simulink model "FBv1_SLOW2DOF"  (R2022b)
settings: Solver=FixedStepAuto  StartTime=0.0  StopTime=Parameter.Time.TMax  FixedStep=Parameter.Time.dt  RelTol=1e-3
values from neighbouring files (symbols this model uses):
  Parameter = DefaultParameter_FBv1_ADv14(Parameter)    [Turbine_Simulation.m]
undefined symbols (not defined in the file or in its folder): x2_t0
libraries: simulink x4
settings Model: LastModifiedBy=felix
settings OptimizationCC: BlockReduction=off  BooleanDataType=off
settings DebuggingCC: SaveWithParameterizedLinksMsg=none  UnderspecifiedInitializationDetection=Classic  MergeDetectMultiDrivingBlocksExec=none  SignalResolutionControl=TryResolveAllWithWarning
settings HardwareCC: TargetUnknown=on
settings ModelReferenceCC: PropagateSignalLabelsOutOfModel=off

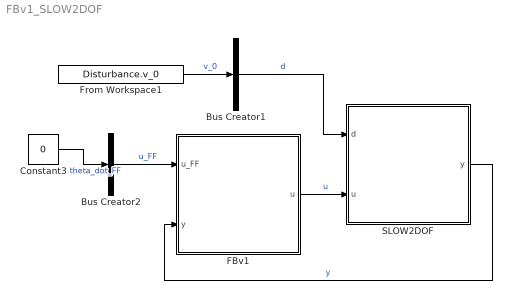
== system FBv1_SLOW2DOF ==
  Bus Creator1 : BusCreator  Inputs=1
  Bus Creator2 : BusCreator  Inputs=1
  Constant3 : Constant  Value=0
  FBv1 : Subsystem
  From Workspace1 : FromWorkspace  VariableName=Disturbance.v_0
  SLOW2DOF : Subsystem
  wires:
  FBv1/1(u) -> SLOW2DOF/2(u)  "u"
  Bus Creator2/1 -> FBv1/1(u_FF)  "u_FF"
  Bus Creator1/1 -> SLOW2DOF/1(d)  "d"
  From Workspace1/1 -> Bus Creator1/1  "v_0"
  SLOW2DOF/1(y) -> FBv1/2(y)  "y"
  Constant3/1 -> Bus Creator2/1  "theta_dot_FF"

== system FBv1_SLOW2DOF/FBv1 ==
  u_FF : Inport
  y : Inport  Port=2
  Bus Creator1 : BusCreator  Inputs=2
  Bus Selector : BusSelector  OutputSignals=Omega_g
  Bus Selector1 : BusSelector  OutputSignals=theta
  Bus Selector2 : BusSelector  OutputSignals=M_g
  FBv1 : Subsystem
  Terminator : Terminator
  u : Outport
  wires:
  y/1 -> Bus Selector2/1, Bus Selector1/1, Bus Selector/1  "y"
  Bus Creator1/1 -> u/1  "u"
  Bus Selector/1 -> FBv1/1(Omega_g [rad/s])  "<Omega_g>"
  u_FF/1 -> Terminator/1
  Bus Selector1/1 -> FBv1/3(theta [rad])  "<theta>"
  FBv1/1(M_g_c [Nm]) -> Bus Creator1/1  "M_g_c"
  FBv1/2(theta_c [rad]) -> Bus Creator1/2  "theta_c"
  Bus Selector2/1 -> FBv1/2(M_g [Nm])  "<M_g>"

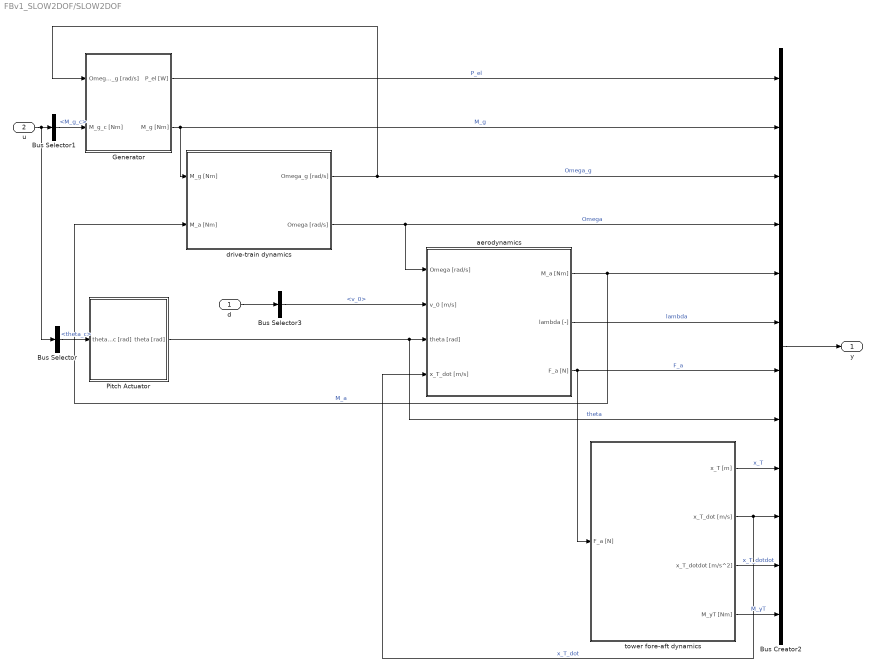
== system FBv1_SLOW2DOF/SLOW2DOF ==
  d : Inport
  u : Inport  Port=2
  Bus Creator2 : BusCreator  Inputs=12
  Bus Selector : BusSelector  OutputSignals=theta_c
  Bus Selector1 : BusSelector  OutputSignals=M_g_c
  Bus Selector3 : BusSelector  OutputSignals=v_0
  Generator : Subsystem
  Pitch Actuator : Subsystem
  "aerodynamics " : Subsystem
  drive-train dynamics : Subsystem
  tower fore-aft dynamics : Subsystem
  y : Outport
  wires:
  Bus Selector3/1 -> "aerodynamics "/2(v_0 [m/s])  "<v_0>"
  d/1 -> Bus Selector3/1
  "aerodynamics "/2(lambda [-]) -> Bus Creator2/6  "lambda"
  Bus Selector/1 -> Pitch Actuator/1(theta_c [rad])  "<theta_c>"
  u/1 -> Bus Selector/1, Bus Selector1/1
  "aerodynamics "/1(M_a [Nm]) -> Bus Creator2/5, drive-train dynamics/2(M_a [Nm])  "M_a"
  drive-train dynamics/2(Omega [rad/s]) -> Bus Creator2/4, "aerodynamics "/1(Omega [rad/s])  "Omega"
  drive-train dynamics/1(Omega_g [rad/s]) -> Bus Creator2/3, Generator/1(Omega_g [rad/s])  "Omega_g"
  Bus Selector1/1 -> Generator/2(M_g_c [Nm])  "<M_g_c>"
  Pitch Actuator/1(theta [rad]) -> Bus Creator2/8, "aerodynamics "/3(theta [rad])  "theta"
  Generator/1(P_el [W]) -> Bus Creator2/1  "P_el"
  Generator/2(M_g [Nm]) -> Bus Creator2/2, drive-train dynamics/1(M_g [Nm])  "M_g"
  "aerodynamics "/3(F_a [N]) -> Bus Creator2/7, tower fore-aft dynamics/1(F_a [N])  "F_a"
  tower fore-aft dynamics/1(x_T [m]) -> Bus Creator2/9  "x_T"
  tower fore-aft dynamics/2(x_T_dot [m/s]) -> "aerodynamics "/4(x_T_dot [m/s]), Bus Creator2/10  "x_T_dot"
  tower fore-aft dynamics/3(x_T_dotdot [m/s^2]) -> Bus Creator2/11  "x_T_dotdot"
  tower fore-aft dynamics/4(M_yT [Nm]) -> Bus Creator2/12  "M_yT"
  Bus Creator2/1 -> y/1

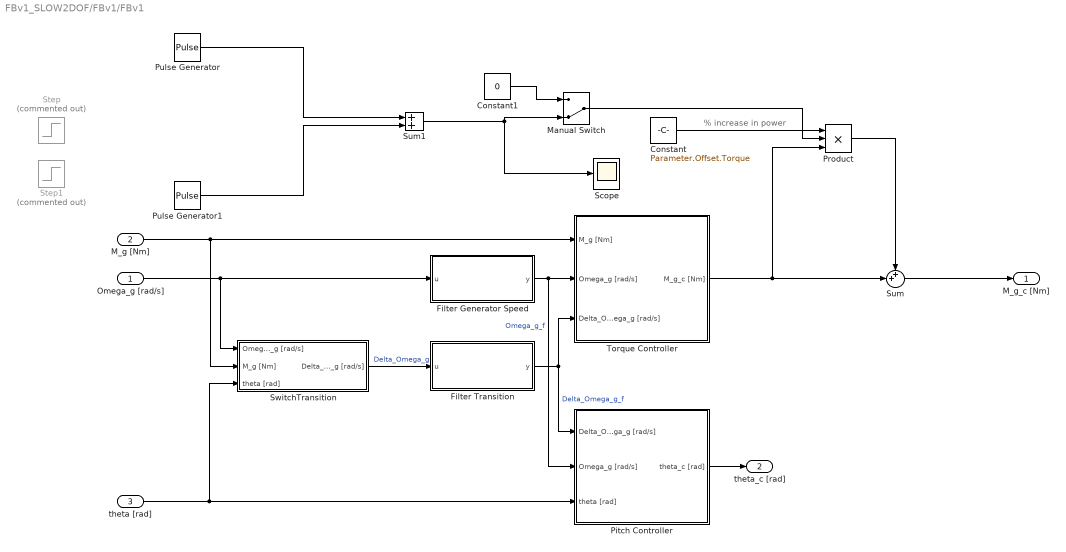
== system FBv1_SLOW2DOF/FBv1/FBv1 ==
  note: % increase in power
  Omega_g [rad/s] : Inport
  M_g [Nm] : Inport  Port=2
  theta [rad] : Inport  Port=3
  Constant : Constant  Value=Parameter.Offset.Torque
  Constant1 : Constant  Value=0
  Filter Generator Speed : Subsystem
  Filter Transition : Subsystem
  Manual Switch : ManualSwitch  CurrentSetting=0
  Pitch Controller : Subsystem
  Product : Product  Inputs=3
  Pulse Generator : DiscretePulseGenerator  PulseType=Time based  Period=Parameter.Offset.positive.period  PulseWidth=Parameter.Offset.positive.width  PhaseDelay=Parameter.Offset.positive.delay
  Pulse Generator1 : DiscretePulseGenerator  PulseType=Time based  Amplitude=-1  Period=Parameter.Offset.negative.period  PulseWidth=Parameter.Offset.negative.width  PhaseDelay=Parameter.Offset.negative.delay
  Scope : Scope
  Step : Step  Commented=on  Time=30  SampleTime=0
  Step1 : Step  Commented=on  Time=32  Before=1  After=0  SampleTime=0
  Sum : Sum  Inputs=++|
  Sum1 : Sum
  SwitchTransition : Subsystem
  Torque Controller : Subsystem
  M_g_c [Nm] : Outport
  theta_c [rad] : Outport  Port=2
  wires:
  Pitch Controller/1(theta_c [rad]) -> theta_c [rad]/1
  Omega_g [rad/s]/1 -> SwitchTransition/1(Omega_g [rad/s]), Filter Generator Speed/1(u)
  SwitchTransition/1(Delta_Omega_g [rad/s]) -> Filter Transition/1(u)  "Delta_Omega_g"
  Filter Transition/1(y) -> Pitch Controller/1(Delta_Omega_g [rad/s]), Torque Controller/3(Delta_Omega_g [rad/s])  "Delta_Omega_g_f"
  Filter Generator Speed/1(y) -> Torque Controller/2(Omega_g [rad/s]), Pitch Controller/2(Omega_g [rad/s])  "Omega_g_f"
  theta [rad]/1 -> Pitch Controller/3(theta [rad]), SwitchTransition/3(theta [rad])
  M_g [Nm]/1 -> SwitchTransition/2(M_g [Nm]), Torque Controller/1(M_g [Nm])
  Torque Controller/1(M_g_c [Nm]) -> Sum/2, Product/3
  Sum/1 -> M_g_c [Nm]/1
  Constant/1 -> Product/1
  Product/1 -> Sum/1
  Manual Switch/1 -> Product/2
  Constant1/1 -> Manual Switch/1
  Sum1/1 -> Scope/1, Manual Switch/2
  Pulse Generator1/1 -> Sum1/2
  Pulse Generator/1 -> Sum1/1

== system FBv1_SLOW2DOF/SLOW2DOF/Generator ==
  Omega_g [rad/s] : Inport
  M_g_c [Nm] : Inport  Port=2
  Constant3 : Constant  Value=Parameter.Generator.eta_el
  Product1 : Product  Inputs=***  RndMeth=Zero
  Simple Torque Actuator : Memory  InitialCondition=Parameter.IC.M_g
  P_el [W] : Outport
  M_g [Nm] : Outport  Port=2
  wires:
  Constant3/1 -> Product1/3
  M_g_c [Nm]/1 -> Simple Torque Actuator/1
  Omega_g [rad/s]/1 -> Product1/2
  Product1/1 -> P_el [W]/1
  Simple Torque Actuator/1 -> M_g [Nm]/1, Product1/1

== system FBv1_SLOW2DOF/SLOW2DOF/Pitch Actuator ==
  theta_c [rad] : Inport
  Constant2 : Constant  Value=Parameter.IC.theta
  PT2 : Subsystem  mask{omega=Parameter.PitchActuator.omega, xi=Parameter.PitchActuator.xi, x1_max=Parameter.PitchActuator.theta_dot_max, x1_min=-Parameter.PitchActuator.theta_dot_max, x2_max=Parameter.PitchActuator.theta_max, x2_min=Parameter.PitchActuator.theta_min}
      mask prompts: omega "undamped natural frequency [rad/s]"; xi "damping factor [-]"; x1_max "Upper bound x1"; x1_min "Lower bound x1"; x2_max "Upper bound x2"; x2_min "Lower bound x2"
      mask Display:
      | disp(['omega = ',num2str(omega),'\n'...
      |     ,'xi = ',num2str(xi)])
      | port_label('output',1,'y')
      | port_label('output',2,'x1')
      | port_label('input',2,'y0')
      | port_label('input',1,'u')
  Terminator : Terminator
  theta [rad] : Outport
  wires:
  theta_c [rad]/1 -> PT2/1(u)
  Constant2/1 -> PT2/2(y0)
  PT2/1(y) -> theta [rad]/1
  PT2/2(x1) -> Terminator/1

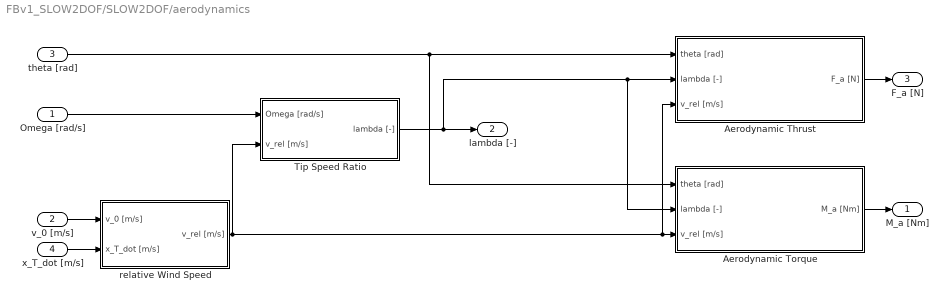
== system FBv1_SLOW2DOF/SLOW2DOF/aerodynamics  ==
  Omega [rad/s] : Inport
  v_0 [m/s] : Inport  Port=2
  theta [rad] : Inport  Port=3
  x_T_dot [m/s] : Inport  Port=4
  Aerodynamic Thrust : Subsystem
  Aerodynamic Torque : Subsystem
  Tip Speed Ratio : Subsystem
  relative Wind Speed : Subsystem
  M_a [Nm] : Outport
  lambda [-] : Outport  Port=2
  F_a [N] : Outport  Port=3
  wires:
  theta [rad]/1 -> Aerodynamic Thrust/1(theta [rad]), Aerodynamic Torque/1(theta [rad])
  Aerodynamic Torque/1(M_a [Nm]) -> M_a [Nm]/1
  Aerodynamic Thrust/1(F_a [N]) -> F_a [N]/1
  x_T_dot [m/s]/1 -> relative Wind Speed/2(x_T_dot [m/s])
  v_0 [m/s]/1 -> relative Wind Speed/1(v_0 [m/s])
  Omega [rad/s]/1 -> Tip Speed Ratio/1(Omega [rad/s])
  relative Wind Speed/1(v_rel [m/s]) -> Tip Speed Ratio/2(v_rel [m/s]), Aerodynamic Torque/3(v_rel [m/s]), Aerodynamic Thrust/3(v_rel [m/s])
  Tip Speed Ratio/1(lambda [-]) -> Aerodynamic Thrust/2(lambda [-]), Aerodynamic Torque/2(lambda [-]), lambda [-]/1

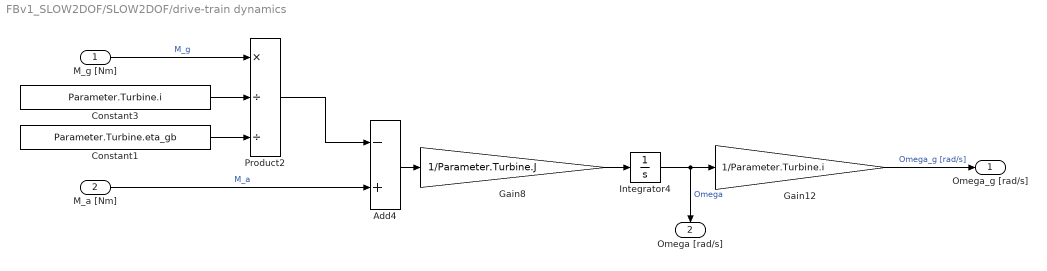
== system FBv1_SLOW2DOF/SLOW2DOF/drive-train dynamics ==
  M_g [Nm] : Inport
  M_a [Nm] : Inport  Port=2
  Add4 : Sum  Inputs=-+
  Constant1 : Constant  Value=Parameter.Turbine.eta_gb
  Constant3 : Constant  Value=Parameter.Turbine.i
  Gain12 : Gain  Gain=1/Parameter.Turbine.i  SaturateOnIntegerOverflow=on  OutDataTypeStr=Inherit: Same as input  ParamDataTypeStr=Inherit: Same as input
  Gain8 : Gain  Gain=1/Parameter.Turbine.J  SaturateOnIntegerOverflow=on  OutDataTypeStr=Inherit: Same as input  ParamDataTypeStr=Inherit: Same as input
  Integrator4 : Integrator  InitialCondition=Parameter.IC.Omega
  Product2 : Product  Inputs=*//  RndMeth=Zero
  Omega_g [rad/s] : Outport
  Omega [rad/s] : Outport  Port=2
  wires:
  M_a [Nm]/1 -> Add4/2  "M_a"
  Integrator4/1 -> Omega [rad/s]/1, Gain12/1  "Omega"
  Add4/1 -> Gain8/1
  Gain8/1 -> Integrator4/1
  Product2/1 -> Add4/1
  Gain12/1 -> Omega_g [rad/s]/1  "Omega_g [rad/s]"
  M_g [Nm]/1 -> Product2/1  "M_g"
  Constant3/1 -> Product2/2
  Constant1/1 -> Product2/3

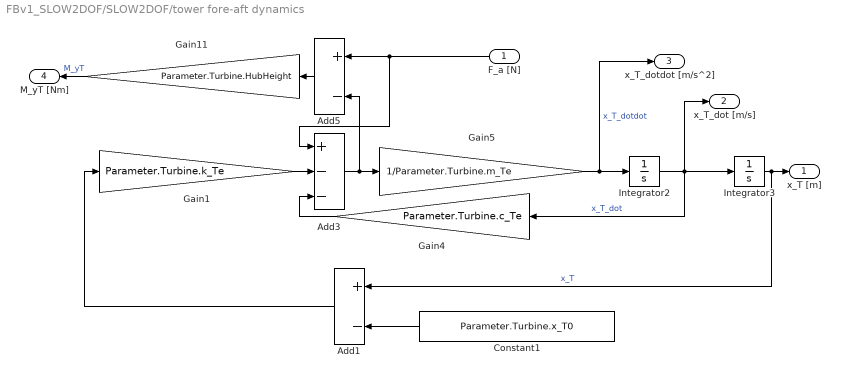
== system FBv1_SLOW2DOF/SLOW2DOF/tower fore-aft dynamics ==
  F_a [N] : Inport
  Add1 : Sum  Inputs=+-
  Add3 : Sum  Inputs=+--
  Add5 : Sum  Inputs=+-
  Constant1 : Constant  Value=Parameter.Turbine.x_T0
  Gain1 : Gain  Gain=Parameter.Turbine.k_Te  SaturateOnIntegerOverflow=on  OutDataTypeStr=Inherit: Same as input  ParamDataTypeStr=Inherit: Same as input
  Gain11 : Gain  Gain=Parameter.Turbine.HubHeight  SaturateOnIntegerOverflow=on  OutDataTypeStr=Inherit: Same as input  ParamDataTypeStr=Inherit: Same as input
  Gain4 : Gain  Gain=Parameter.Turbine.c_Te  SaturateOnIntegerOverflow=on  OutDataTypeStr=Inherit: Same as input  ParamDataTypeStr=Inherit: Same as input
  Gain5 : Gain  Gain=1/Parameter.Turbine.m_Te  SaturateOnIntegerOverflow=on  OutDataTypeStr=Inherit: Same as input  ParamDataTypeStr=Inherit: Same as input
  Integrator2 : Integrator
  Integrator3 : Integrator  InitialCondition=Parameter.IC.x_T
  x_T [m] : Outport
  x_T_dot [m/s] : Outport  Port=2
  x_T_dotdot [m/s^2] : Outport  Port=3
  M_yT [Nm] : Outport  Port=4
  wires:
  Constant1/1 -> Add1/2
  Add1/1 -> Gain1/1
  Add3/1 -> Gain5/1, Add5/2
  Integrator2/1 -> Gain4/1, Integrator3/1, x_T_dot [m/s]/1  "x_T_dot"
  Integrator3/1 -> x_T [m]/1, Add1/1  "x_T"
  Gain4/1 -> Add3/3
  Gain1/1 -> Add3/2
  Gain5/1 -> x_T_dotdot [m/s^2]/1, Integrator2/1  "x_T_dotdot"
  Add5/1 -> Gain11/1
  Gain11/1 -> M_yT [Nm]/1  "M_yT"
  F_a [N]/1 -> Add5/1, Add3/1

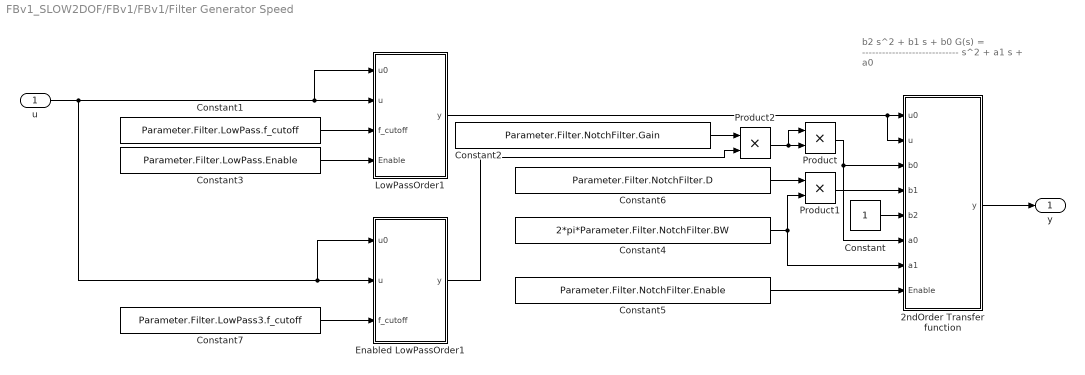
== system FBv1_SLOW2DOF/FBv1/FBv1/Filter Generator Speed ==
  note: b2 s^2 + b1 s + b0
      | G(s) = -----------------------------
      | s^2 + a1 s + a0
  u : Inport
  2ndOrder Transfer function : Subsystem
  Constant : Constant
  Constant1 : Constant  Value=Parameter.Filter.LowPass.f_cutoff
  Constant2 : Constant  Value=Parameter.Filter.NotchFilter.Gain
  Constant3 : Constant  Value=Parameter.Filter.LowPass.Enable
  Constant4 : Constant  Value=2*pi*Parameter.Filter.NotchFilter.BW
  Constant5 : Constant  Value=Parameter.Filter.NotchFilter.Enable
  Constant6 : Constant  Value=Parameter.Filter.NotchFilter.D
  Constant7 : Constant  Value=Parameter.Filter.LowPass3.f_cutoff
  Enabled LowPassOrder1 : Subsystem
  LowPassOrder1 : Subsystem
  Product : Product  RndMeth=Zero
  Product1 : Product  RndMeth=Zero
  Product2 : Product  RndMeth=Zero
  y : Outport
  wires:
  u/1 -> LowPassOrder1/1(u0), LowPassOrder1/2(u), Enabled LowPassOrder1/1(u0), Enabled LowPassOrder1/2(u)
  Constant3/1 -> LowPassOrder1/4(Enable)
  Constant1/1 -> LowPassOrder1/3(f_cutoff)
  LowPassOrder1/1(y) -> 2ndOrder Transfer function/2(u), 2ndOrder Transfer function/1(u0)
  Constant5/1 -> 2ndOrder Transfer function/8(Enable)
  Product/1 -> 2ndOrder Transfer function/3(b0), 2ndOrder Transfer function/6(a0)
  Product2/1 -> Product/1, Product/2
  Product1/1 -> 2ndOrder Transfer function/4(b1)
  Constant6/1 -> Product1/1
  Constant4/1 -> 2ndOrder Transfer function/7(a1), Product1/2
  2ndOrder Transfer function/1(y) -> y/1
  Constant/1 -> 2ndOrder Transfer function/5(b2)
  Constant7/1 -> Enabled LowPassOrder1/3(f_cutoff)
  Constant2/1 -> Product2/1
  Enabled LowPassOrder1/1(y) -> Product2/2

== system FBv1_SLOW2DOF/FBv1/FBv1/Filter Transition ==
  u : Inport
  Constant1 : Constant  Value=Parameter.Filter.LowPass2.f_cutoff
  Dummy : Constant  Value=0
  LowPassOrder1 : Subsystem
  y : Outport
  wires:
  LowPassOrder1/1(y) -> y/1
  u/1 -> LowPassOrder1/2(u)
  Constant1/1 -> LowPassOrder1/3(f_cutoff)
  Dummy/1 -> LowPassOrder1/1(u0)

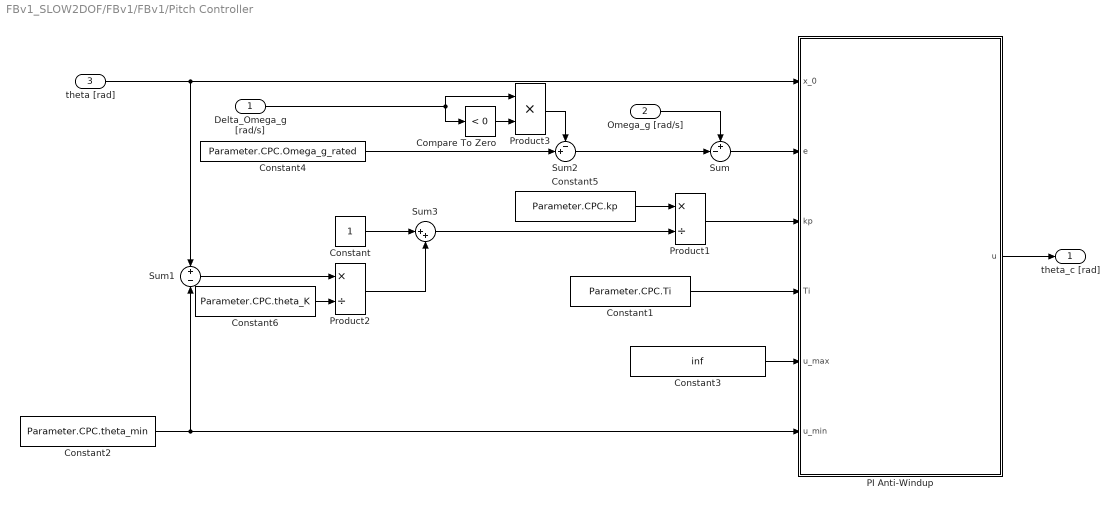
== system FBv1_SLOW2DOF/FBv1/FBv1/Pitch Controller ==
  Delta_Omega_g [rad/s] : Inport
  Omega_g [rad/s] : Inport  Port=2
  theta [rad] : Inport  Port=3
  Compare To Zero : simulink/Logic and Bit Operations/Compare To Zero  relop=<  OutDataTypeStr=boolean
  Constant : Constant
  Constant1 : Constant  Value=Parameter.CPC.Ti
  Constant2 : Constant  Value=Parameter.CPC.theta_min
  Constant3 : Constant  Value=inf
  Constant4 : Constant  Value=Parameter.CPC.Omega_g_rated
  Constant5 : Constant  Value=Parameter.CPC.kp
  Constant6 : Constant  Value=Parameter.CPC.theta_K
  PI Anti-Windup : Subsystem
  Product1 : Product  Inputs=*/
  Product2 : Product  Inputs=*/
  Product3 : Product
  Sum : Sum  Inputs=+-|
  Sum1 : Sum  Inputs=+|-
  Sum2 : Sum  Inputs=-+|
  Sum3 : Sum  Inputs=|++
  theta_c [rad] : Outport
  wires:
  Product1/1 -> PI Anti-Windup/3(kp)
  theta [rad]/1 -> PI Anti-Windup/1(x_0), Sum1/1
  Sum/1 -> PI Anti-Windup/2(e)
  PI Anti-Windup/1(u) -> theta_c [rad]/1
  Constant2/1 -> PI Anti-Windup/6(u_min), Sum1/2
  Delta_Omega_g [rad/s]/1 -> Product3/1, Compare To Zero/1
  Compare To Zero/1 -> Product3/2
  Product3/1 -> Sum2/1
  Constant4/1 -> Sum2/2
  Constant1/1 -> PI Anti-Windup/4(Ti)
  Sum2/1 -> Sum/2
  Omega_g [rad/s]/1 -> Sum/1
  Constant3/1 -> PI Anti-Windup/5(u_max)
  Sum1/1 -> Product2/1
  Constant6/1 -> Product2/2
  Constant/1 -> Sum3/1
  Product2/1 -> Sum3/2
  Constant5/1 -> Product1/1
  Sum3/1 -> Product1/2

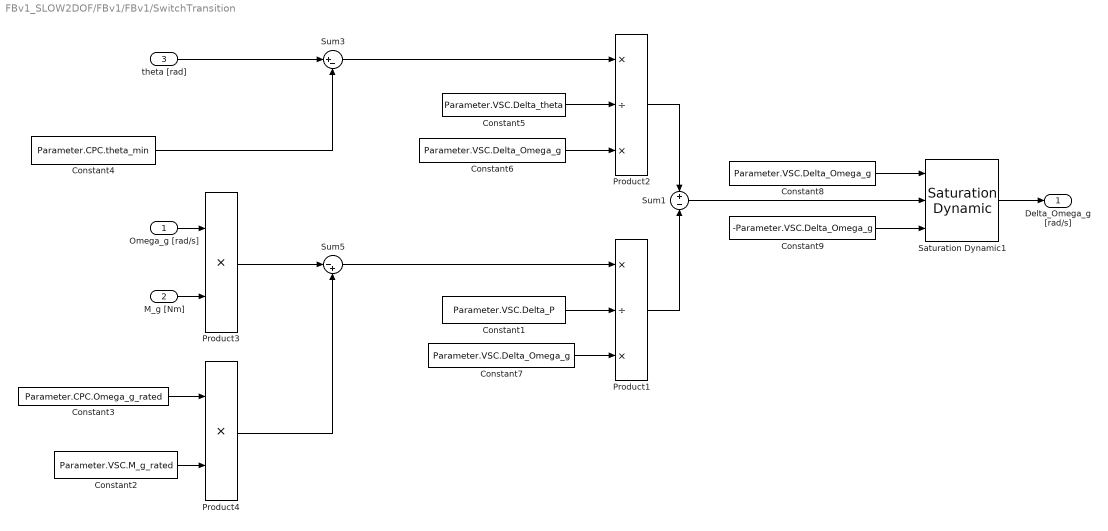
== system FBv1_SLOW2DOF/FBv1/FBv1/SwitchTransition ==
  Omega_g [rad/s] : Inport
  M_g [Nm] : Inport  Port=2
  theta [rad] : Inport  Port=3
  Constant1 : Constant  Value=Parameter.VSC.Delta_P
  Constant2 : Constant  Value=Parameter.VSC.M_g_rated
  Constant3 : Constant  Value=Parameter.CPC.Omega_g_rated
  Constant4 : Constant  Value=Parameter.CPC.theta_min
  Constant5 : Constant  Value=Parameter.VSC.Delta_theta
  Constant6 : Constant  Value=Parameter.VSC.Delta_Omega_g
  Constant7 : Constant  Value=Parameter.VSC.Delta_Omega_g
  Constant8 : Constant  Value=Parameter.VSC.Delta_Omega_g
  Constant9 : Constant  Value=-Parameter.VSC.Delta_Omega_g
  Product1 : Product  Inputs=*/*  RndMeth=Zero
  Product2 : Product  Inputs=*/*  RndMeth=Zero
  Product3 : Product  RndMeth=Zero
  Product4 : Product  RndMeth=Zero
  Saturation Dynamic1 : simulink/Discontinuities/Saturation Dynamic  OutMin=[]  OutMax=[]  OutDataTypeStr=Inherit: Same as second input  OutDataType=fixdt(1, 16)  OutScaling=2^-10  DoSatur=off
  Sum1 : Sum  Inputs=+|-
  Sum3 : Sum  Inputs=|+-
  Sum5 : Sum  Inputs=|-+
  Delta_Omega_g [rad/s] : Outport
  wires:
  theta [rad]/1 -> Sum3/1
  Sum3/1 -> Product2/1
  Product2/1 -> Sum1/1
  Constant5/1 -> Product2/2
  Constant4/1 -> Sum3/2
  Sum5/1 -> Product1/1
  Product1/1 -> Sum1/2
  M_g [Nm]/1 -> Product3/2
  Omega_g [rad/s]/1 -> Product3/1
  Product3/1 -> Sum5/1
  Constant2/1 -> Product4/2
  Constant3/1 -> Product4/1
  Product4/1 -> Sum5/2
  Constant6/1 -> Product2/3
  Constant1/1 -> Product1/2
  Constant7/1 -> Product1/3
  Saturation Dynamic1/1 -> Delta_Omega_g [rad/s]/1
  Sum1/1 -> Saturation Dynamic1/2
  Constant8/1 -> Saturation Dynamic1/1
  Constant9/1 -> Saturation Dynamic1/3

== system FBv1_SLOW2DOF/FBv1/FBv1/Torque Controller ==
  M_g [Nm] : Inport
  Omega_g [rad/s] : Inport  Port=2
  Delta_Omega_g [rad/s] : Inport  Port=3
  Constant : Constant  Value=Parameter.VSC.kp
  Constant1 : Constant  Value=Parameter.VSC.Ti
  LimitsAndReferenceValueTC : Subsystem
  PI Anti-Windup : Subsystem
  Sum : Sum  Inputs=|+-
  M_g_c [Nm] : Outport
  wires:
  LimitsAndReferenceValueTC/1(Omega_g_ref [rad/s]) -> Sum/2
  M_g [Nm]/1 -> PI Anti-Windup/1(x_0)
  Sum/1 -> PI Anti-Windup/2(e)
  Constant/1 -> PI Anti-Windup/3(kp)
  Constant1/1 -> PI Anti-Windup/4(Ti)
  Omega_g [rad/s]/1 -> LimitsAndReferenceValueTC/1(Omega_g [rad/s]), Sum/1
  LimitsAndReferenceValueTC/2(M_g_ub [Nm]) -> PI Anti-Windup/5(u_max)  "M_g_ub"
  LimitsAndReferenceValueTC/3(M_g_lb [Nm]) -> PI Anti-Windup/6(u_min)  "M_g_lb"
  PI Anti-Windup/1(u) -> M_g_c [Nm]/1
  Delta_Omega_g [rad/s]/1 -> LimitsAndReferenceValueTC/2(Delta_Omega_g [rad/s])

== system FBv1_SLOW2DOF/SLOW2DOF/Pitch Actuator/PT2 ==
  u : Inport
  y0 : Inport  Port=2
  Add3 : Sum  Inputs=+--
  Gain1 : Gain  Gain=omega*omega  SaturateOnIntegerOverflow=on  OutDataTypeStr=Inherit: Same as input  ParamDataTypeStr=Inherit: Same as input
  Gain2 : Gain  Gain=omega*omega  SaturateOnIntegerOverflow=on  OutDataTypeStr=Inherit: Same as input  ParamDataTypeStr=Inherit: Same as input
  Gain3 : Gain  Gain=2*xi*omega  SaturateOnIntegerOverflow=on  OutDataTypeStr=Inherit: Same as input  ParamDataTypeStr=Inherit: Same as input
  Integrator1 : Integrator  LimitOutput=on  UpperSaturationLimit=x1_max  LowerSaturationLimit=x1_min
  Integrator2 : Integrator  InitialConditionSource=external  InitialCondition=x2_t0  LimitOutput=on  UpperSaturationLimit=x2_max  LowerSaturationLimit=x2_min
  y : Outport
  x1 : Outport  Port=2
  wires:
  Gain3/1 -> Add3/3
  u/1 -> Gain1/1
  Add3/1 -> Integrator1/1
  Gain1/1 -> Add3/1
  Gain2/1 -> Add3/2
  Integrator1/1 -> x1/1, Gain3/1, Integrator2/1  "x1"
  y0/1 -> Integrator2/2
  Integrator2/1 -> Gain2/1, y/1

== system FBv1_SLOW2DOF/SLOW2DOF/aerodynamics /Aerodynamic Thrust ==
  theta [rad] : Inport
  lambda [-] : Inport  Port=2
  v_rel [m/s] : Inport  Port=3
  Fcn1 : Fcn  Expr=1/2*Parameter.General.rho*pi*Parameter.Turbine.R^2*u(1)
  Product1 : Product  Inputs=3  RndMeth=Zero
  effective force coefficient : Lookup2D  RowIndex=Parameter.Turbine.SS.lambda  ColumnIndex=Parameter.Turbine.SS.theta  Table=Parameter.Turbine.SS.c_T  SaturateOnIntegerOverflow=off  InputSameDT=off
  F_a [N] : Outport
  wires:
  v_rel [m/s]/1 -> Product1/2, Product1/1
  theta [rad]/1 -> effective force coefficient/2
  lambda [-]/1 -> effective force coefficient/1
  Fcn1/1 -> Product1/3
  Product1/1 -> F_a [N]/1  "F_a"
  effective force coefficient/1 -> Fcn1/1  "c_T"

== system FBv1_SLOW2DOF/SLOW2DOF/aerodynamics /Aerodynamic Torque ==
  theta [rad] : Inport
  lambda [-] : Inport  Port=2
  v_rel [m/s] : Inport  Port=3
  Fcn1 : Fcn  Expr=1/2*Parameter.General.rho*pi*Parameter.Turbine.R^3*u(1)
  Product1 : Product  Inputs=3  RndMeth=Zero
  Product2 : Product  Inputs=/*  RndMeth=Zero
  effective power coefficient : Lookup2D  RowIndex=Parameter.Turbine.SS.lambda  ColumnIndex=Parameter.Turbine.SS.theta  Table=Parameter.Turbine.SS.c_P  SaturateOnIntegerOverflow=off  InputSameDT=off
  M_a [Nm] : Outport
  wires:
  Product1/1 -> M_a [Nm]/1  "M_a"
  Fcn1/1 -> Product1/3
  lambda [-]/1 -> effective power coefficient/1, Product2/1
  theta [rad]/1 -> effective power coefficient/2
  v_rel [m/s]/1 -> Product1/1, Product1/2
  effective power coefficient/1 -> Product2/2  "c_P"
  Product2/1 -> Fcn1/1

== system FBv1_SLOW2DOF/SLOW2DOF/aerodynamics /Tip Speed Ratio ==
  Omega [rad/s] : Inport
  v_rel [m/s] : Inport  Port=2
  Gain6 : Gain  Gain=Parameter.Turbine.R  SaturateOnIntegerOverflow=on  OutDataTypeStr=Inherit: Same as input  ParamDataTypeStr=Inherit: Same as input
  Product3 : Product  Inputs=*/  RndMeth=Zero
  lambda [-] : Outport
  wires:
  Product3/1 -> Gain6/1
  Omega [rad/s]/1 -> Product3/1
  v_rel [m/s]/1 -> Product3/2
  Gain6/1 -> lambda [-]/1  "lambda"

== system FBv1_SLOW2DOF/SLOW2DOF/aerodynamics /relative Wind Speed ==
  v_0 [m/s] : Inport
  x_T_dot [m/s] : Inport  Port=2
  Add2 : Sum  Inputs=-+
  v_rel [m/s] : Outport
  wires:
  Add2/1 -> v_rel [m/s]/1  "v_rel"
  x_T_dot [m/s]/1 -> Add2/1
  v_0 [m/s]/1 -> Add2/2

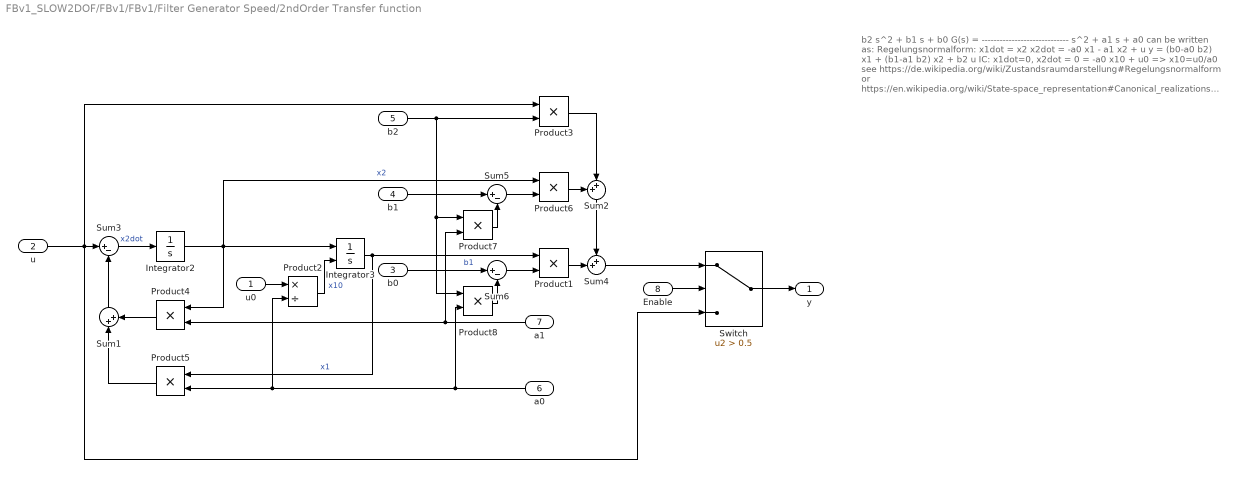
== system FBv1_SLOW2DOF/FBv1/FBv1/Filter Generator Speed/2ndOrder Transfer function ==
  note: b2 s^2 + b1 s + b0
      | G(s) = -----------------------------
      | s^2 + a1 s + a0
      |
      | can be written as:
      |
      | Regelungsnormalform:
      | x1dot = x2
      | x2dot = -a0 x1 - a1 x2 + u
      | y = (b0-a0 b2) x1 + (b1-a1 b2) x2 + b2 u
      |
      | IC: x1dot=0, x2dot = 0 = -a0 x10 + u0 => x10=u0/a0
      |
      | see https://de.wikipedia.org/wiki/Zustandsraumdarstellung#Regelungsnormalform
      | or
      | https://en.wikipedia.org/wiki/State-space_representation#Canonical_realizations
      |
      | Advantage:
      | - IC can be set
      | - coefficients can be changed online
  u0 : Inport
  u : Inport  Port=2
  b0 : Inport  Port=3
  b1 : Inport  Port=4
  b2 : Inport  Port=5
  a0 : Inport  Port=6
  a1 : Inport  Port=7
  Enable : Inport  Port=8
  Integrator2 : Integrator
  Integrator3 : Integrator  InitialConditionSource=external
  Product{1,3..8} (7 alike) : Product  RndMeth=Zero
  Product2 : Product  Inputs=*/  RndMeth=Zero
  Sum1 : Sum  Inputs=|++
  Sum2 : Sum  Inputs=++|
  Sum3 : Sum  Inputs=|+-
  Sum4 : Sum  Inputs=++|
  Sum5 : Sum  Inputs=|+-
  Sum6 : Sum  Inputs=|+-
  Switch : Switch  Criteria=u2 > Threshold  Threshold=0.5  SaturateOnIntegerOverflow=off  InputSameDT=off
  y : Outport
  wires:
  Switch/1 -> y/1
  Enable/1 -> Switch/2
  Integrator2/1 -> Integrator3/1, Product6/1, Product4/1  "x2"
  Integrator3/1 -> Product1/1, Product5/1  "x1"
  Sum3/1 -> Integrator2/1  "x2dot"
  u/1 -> Product3/1, Sum3/1, Switch/3
  Sum4/1 -> Switch/1
  Product1/1 -> Sum4/2
  Product6/1 -> Sum2/1
  Sum2/1 -> Sum4/1
  Sum1/1 -> Sum3/2
  Product4/1 -> Sum1/2
  Product5/1 -> Sum1/1
  a0/1 -> Product8/2, Product2/2, Product5/2
  a1/1 -> Product7/2, Product4/2
  b2/1 -> Product8/1, Product7/1, Product3/2
  Product3/1 -> Sum2/2
  Sum5/1 -> Product6/2
  b1/1 -> Sum5/1
  Product7/1 -> Sum5/2
  Sum6/1 -> Product1/2
  b0/1 -> Sum6/1  "b1"
  Product8/1 -> Sum6/2
  Product2/1 -> Integrator3/2  "x10"
  u0/1 -> Product2/1

== system FBv1_SLOW2DOF/FBv1/FBv1/Filter Generator Speed/Enabled LowPassOrder1 ==
  u0 : Inport
  u : Inport  Port=2
  f_cutoff : Inport  Port=3
  Add3 : Sum  Inputs=-+
  Integrator : Integrator  InitialConditionSource=external
  Product : Product  Inputs=3  RndMeth=Zero
  hz to rad : Constant  Value=2*pi
  y : Outport
  wires:
  u0/1 -> Integrator/2
  Integrator/1 -> y/1, Add3/1
  u/1 -> Add3/2
  Product/1 -> Integrator/1
  Add3/1 -> Product/3
  f_cutoff/1 -> Product/2
  hz to rad/1 -> Product/1

== system FBv1_SLOW2DOF/FBv1/FBv1/Filter Generator Speed/LowPassOrder1 ==
  u0 : Inport
  u : Inport  Port=2
  f_cutoff : Inport  Port=3
  Enable : Inport  Port=4
  Add3 : Sum  Inputs=-+
  Integrator : Integrator  InitialConditionSource=external
  Product : Product  Inputs=3  RndMeth=Zero
  Switch : Switch  Criteria=u2 > Threshold  Threshold=0.5  SaturateOnIntegerOverflow=off  InputSameDT=off
  hz to rad : Constant  Value=2*pi
  y : Outport
  wires:
  u0/1 -> Integrator/2
  Switch/1 -> y/1
  Enable/1 -> Switch/2
  u/1 -> Add3/2, Switch/3
  Integrator/1 -> Switch/1, Add3/1
  Product/1 -> Integrator/1
  Add3/1 -> Product/3
  f_cutoff/1 -> Product/2
  hz to rad/1 -> Product/1

== system FBv1_SLOW2DOF/FBv1/FBv1/Filter Transition/LowPassOrder1 ==
  u0 : Inport
  u : Inport  Port=2
  f_cutoff : Inport  Port=3
  Add3 : Sum  Inputs=-+
  Integrator : Integrator  InitialConditionSource=external
  Product : Product  Inputs=3  RndMeth=Zero
  hz to rad : Constant  Value=2*pi
  y : Outport
  wires:
  u0/1 -> Integrator/2
  Integrator/1 -> y/1, Add3/1
  u/1 -> Add3/2
  Product/1 -> Integrator/1
  Add3/1 -> Product/3
  f_cutoff/1 -> Product/2
  hz to rad/1 -> Product/1

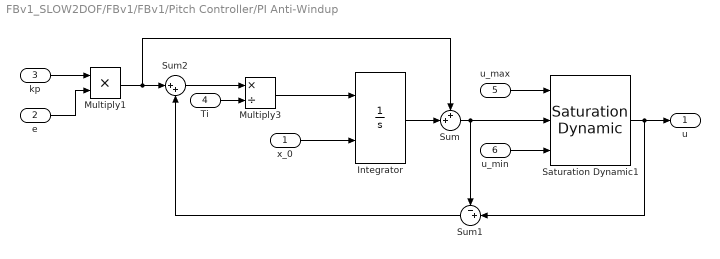
== system FBv1_SLOW2DOF/FBv1/FBv1/Pitch Controller/PI Anti-Windup ==
  x_0 : Inport
  e : Inport  Port=2
  kp : Inport  Port=3
  Ti : Inport  Port=4
  u_max : Inport  Port=5
  u_min : Inport  Port=6
  Integrator : Integrator  InitialConditionSource=external
  Multiply1 : Product  Inputs=**
  Multiply3 : Product  Inputs=*/
  Saturation Dynamic1 : simulink/Discontinuities/Saturation Dynamic  OutMin=[]  OutMax=[]  OutDataTypeStr=Inherit: Same as second input  OutDataType=fixdt(1, 16)  OutScaling=2^-10  DoSatur=off
  Sum : Sum  Inputs=++|
  Sum1 : Sum  Inputs=-+|
  Sum2 : Sum  Inputs=|++
  u : Outport
  wires:
  Saturation Dynamic1/1 -> u/1, Sum1/2
  Integrator/1 -> Sum/2
  kp/1 -> Multiply1/1
  e/1 -> Multiply1/2
  Ti/1 -> Multiply3/2
  Sum1/1 -> Sum2/2
  Multiply1/1 -> Sum/1, Sum2/1
  Sum2/1 -> Multiply3/1
  x_0/1 -> Integrator/2
  Multiply3/1 -> Integrator/1
  u_min/1 -> Saturation Dynamic1/3
  Sum/1 -> Saturation Dynamic1/2, Sum1/1
  u_max/1 -> Saturation Dynamic1/1

== system FBv1_SLOW2DOF/FBv1/FBv1/Torque Controller/LimitsAndReferenceValueTC ==
  Omega_g [rad/s] : Inport
  Delta_Omega_g [rad/s] : Inport  Port=2
  Constant1 : Constant  Value=Parameter.VSC.Omega_g_1d5
  Constant2 : Constant  Value=Parameter.VSC.M_g_rated
  Constant3 : Constant  Value=Parameter.VSC.k
  Constant5 : Constant  Value=Parameter.CPC.Omega_g_rated
  Constant6 : Constant  Value=Parameter.VSC.i_G_max
  LimitsAndReferenceValueTC : MATLAB Function  TreatAsAtomicUnit=on
  Omega_g_ref [rad/s] : Outport
  M_g_ub [Nm] : Outport  Port=2
  M_g_lb [Nm] : Outport  Port=3
  wires:
  LimitsAndReferenceValueTC/2(M_g_ub) -> M_g_ub [Nm]/1  "M_g_ub"
  Omega_g [rad/s]/1 -> LimitsAndReferenceValueTC/1(Omega_g)
  Constant1/1 -> LimitsAndReferenceValueTC/3(Omega_g_1d5)
  Constant3/1 -> LimitsAndReferenceValueTC/4(k)
  Constant2/1 -> LimitsAndReferenceValueTC/6(M_g_rated)
  Constant5/1 -> LimitsAndReferenceValueTC/5(Omega_g_rated)
  LimitsAndReferenceValueTC/1(Omega_g_ref) -> Omega_g_ref [rad/s]/1  "Omega_g_ref"
  LimitsAndReferenceValueTC/3(M_g_lb) -> M_g_lb [Nm]/1  "M_g_lb"
  Constant6/1 -> LimitsAndReferenceValueTC/7(i_G_max)
  Delta_Omega_g [rad/s]/1 -> LimitsAndReferenceValueTC/2(Delta_Omega_g)

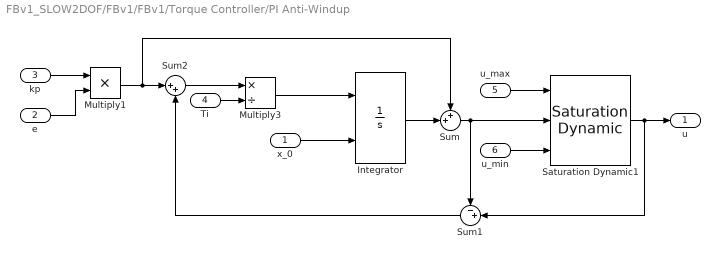
== system FBv1_SLOW2DOF/FBv1/FBv1/Torque Controller/PI Anti-Windup ==
  x_0 : Inport
  e : Inport  Port=2
  kp : Inport  Port=3
  Ti : Inport  Port=4
  u_max : Inport  Port=5
  u_min : Inport  Port=6
  Integrator : Integrator  InitialConditionSource=external
  Multiply1 : Product  Inputs=**
  Multiply3 : Product  Inputs=*/
  Saturation Dynamic1 : simulink/Discontinuities/Saturation Dynamic  OutMin=[]  OutMax=[]  OutDataTypeStr=Inherit: Same as second input  OutDataType=fixdt(1, 16)  OutScaling=2^-10  DoSatur=off
  Sum : Sum  Inputs=++|
  Sum1 : Sum  Inputs=-+|
  Sum2 : Sum  Inputs=|++
  u : Outport
  wires:
  Saturation Dynamic1/1 -> u/1, Sum1/2
  Integrator/1 -> Sum/2
  kp/1 -> Multiply1/1
  e/1 -> Multiply1/2
  Ti/1 -> Multiply3/2
  Sum1/1 -> Sum2/2
  Multiply1/1 -> Sum/1, Sum2/1
  Sum2/1 -> Multiply3/1
  x_0/1 -> Integrator/2
  Multiply3/1 -> Integrator/1
  u_min/1 -> Saturation Dynamic1/3
  Sum/1 -> Saturation Dynamic1/2, Sum1/1
  u_max/1 -> Saturation Dynamic1/1

== matlab function FBv1_SLOW2DOF/FBv1/FBv1/Torque Controller/LimitsAndReferenceValueTC/LimitsAndReferenceValueTC ==
  settings: fimath=|
      | fimath(...
      | 'RoundMode', 'floor',...
      | 'OverflowMode', 'wrap',...
      | 'ProductMode', 'KeepLSB', 'ProductWordLength', 32,...
      | 'SumMode', 'KeepLSB', 'SumWordLength', 32,...
      | 'CastBeforeSum', false)
  data: Omega_g_ref output; M_g_ub output; M_g_lb output; Omega_g input; Delta_Omega_g input; Omega_g_1d5 input; k input; Omega_g_rated input; M_g_rated input; i_G_max input
function [Omega_g_ref,M_g_ub,M_g_lb] = LimitsAndReferenceValueTC(...
    Omega_g,Delta_Omega_g,...               % signals
    Omega_g_1d5,...                         % Region 1.5 parameters
    k,...                                   % Region   2 parameters
    Omega_g_rated,...                       % Region 2.5 parameters
    M_g_rated,...                           % Region   3 parameters
    i_G_max)                                % limits
 


%% Internals
Omega_g_R2Switch    = (Omega_g_1d5+Omega_g_rated)/2;

%% State Machine
if Omega_g<Omega_g_R2Switch
    Omega_g_ref             = Omega_g_1d5;
	M_g_lb                  = 0;
    M_g_ub                  = k*Omega_g^2;
else  
    if Delta_Omega_g<0
        Omega_g_ref     	= Omega_g_rated;
        M_g_lb            	= k*Omega_g^2;
        M_g_ub           	= min(M_g_rated*Omega_g_rated/Omega_g,M_g_rated*i_G_max);
    else
        Omega_g_ref         = Omega_g_rated-Delta_Omega_g;
        M_g_lb              = k*Omega_g^2;
        M_g_ub              = min(M_g_rated*Omega_g_rated/Omega_g,M_g_rated*i_G_max);
    end       
end

end
